simulink model "TrafficLights"  (R2024b)
settings: Solver=VariableStepAuto  StartTime=0.0  StopTime=20  RelTol=1e-3
settings Model: Creator=MOHAMED  LastModifiedBy=MOHAMED

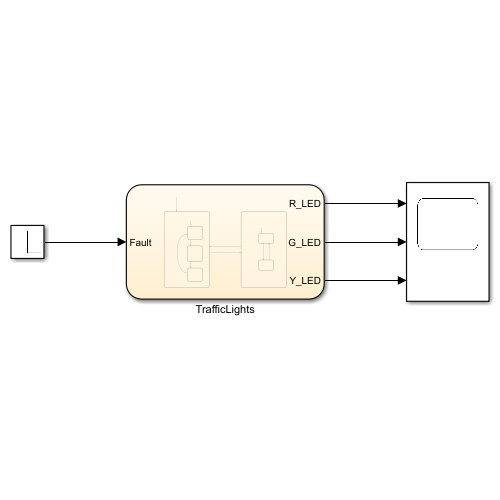
[thumbnail: Simulink's stored preview of the top-level diagram]
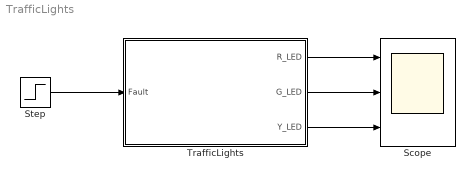
== system TrafficLights ==
  Scope : Scope  NumInputPorts=3
  Step : Step  Time=10  Before=1  After=0  SampleTime=0
  TrafficLights : Stateflow chart  TreatAsAtomicUnit=on
  wires:
  TrafficLights/1(R_LED) -> Scope/1
  Step/1 -> TrafficLights/1(Fault)
  TrafficLights/2(G_LED) -> Scope/2
  TrafficLights/3(Y_LED) -> Scope/3

== stateflow chart TrafficLights/TrafficLights ==
  state NormalMode
    state Stop
      en:
      R_LED = 1;
      ex:
      R_LED = 0;
    state GO
      en:
      G_LED = 1;
      ex:
      G_LED = 0;
    state PTS
      en:
      Y_LED = 1;
      ex:
      Y_LED = 0;
    (default) -> Stop
    PTS -> Stop : after(1, sec)
    Stop -> GO : after(1, sec)
    GO -> PTS : after(1, sec)
  state FaultMode
    state OFF
      en:
      R_LED = 0;
    state ON
      en:
      R_LED = 1;
    (default) -> OFF
    OFF -> ON : after(1, sec)
    ON -> OFF : after(1, sec)
  (default) -> NormalMode
  FaultMode -> NormalMode : [Fault == 0]
  NormalMode -> FaultMode : [Fault == 1]
  data: R_LED output double; G_LED output double; Y_LED output double; Fault input double
